simulink model "arduino_sw_harness"  (R2013b)
settings: Solver=FixedStepDiscrete  SolverMode=SingleTasking  StartTime=0.0  StopTime=10.0  FixedStep=0.1  RelTol=1e-3
libraries: arduinolib x3, simulink x1, sw_lib x1
settings Model: ExtModeTrigDuration=2  Creator=raarenst  LastModifiedBy=raarenst
settings OptimizationCC: OptimizeModelRefInitCode=on  LifeSpan=1
settings DebuggingCC: SolverPrmCheckMsg=none  ParameterPrecisionLossMsg=none
settings HardwareCC: ProdBitPerInt=16  ProdBitPerPointer=8  ProdIntDivRoundTo=Zero  ProdEndianess=LittleEndian  ProdWordSize=8  ProdHWDeviceType=Atmel->AVR
settings RTWCC: SystemTargetFile=realtime.tlc  GenerateMakefile=off  TemplateMakefile=realtime.tmf  Description=Run on Target Hardware  RTWVerbose=off  ProcessScript=realtime_make_rtw_hook
settings STFCustomTargetCC: TargetLibSuffix=.a  GenerateSampleERTMain=on  ERTCustomFileBanners=on  SupportNonInlinedSFcns=off  SupportVariableSizeSignals=on  MATLABClassNameForMDSCustomization=Simulink.SoftwareTarget.ERTCustomization  GRTInterface=off  SystemTargetFile=realtime.tlc
settings ERTTargetCC: CodeReplacementLibrary=ANSI_C  GenerateSampleERTMain=on  ParMdlRefBuildCompliant=off  CompOptLevelCompliant=off  ConcurrentExecutionCompliant=off  CombineOutputUpdateFcns=off  ERTFirstTimeCompliant=off  SupportContinuousTime=on  SupportVariableSizeSignals=on  ModelStepFunctionPrototypeControlCompliant=off  CPPClassGenCompliant=off  ExtModeTransport=3  ExtModeMexFile=ext_serial_win32_comm  ExtModeMexArgs=0 1 9600  InlinedParameterPlacement=NonHierarchical  ERTSrcFileBannerTemplate=realtime_code_template.cgt  ERTHdrFileBannerTemplate=realtime_code_template.cgt  ERTDataSrcFileTemplate=realtime_code_template.cgt  ERTDataHdrFileTemplate=realtime_code_template.cgt  ERTCustomFileTemplate=realtime_file_process.tlc
settings ConfigurationSet: Description=SimMechanics 2G

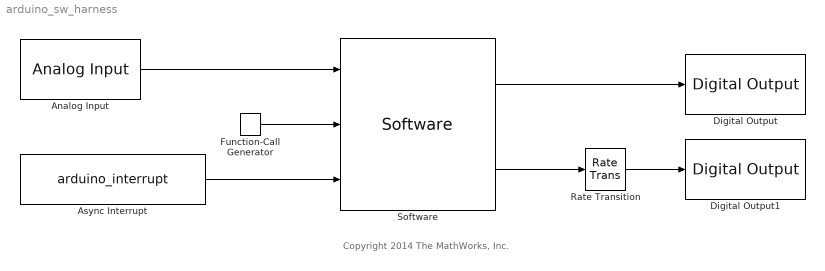
== system arduino_sw_harness ==
  note: Copyright 2014 The MathWorks, Inc.
  Analog Input : arduinolib/Analog Input  pinNumber=0  sampleTime=0.1
  Async Interrupt : S-Function  FunctionName=arduino_interrupt  Parameters=pin_number, int_number, int_mode, show_inputport  EnableBusSupport=off  mask(Arduino Interrupt Block){int_number=0, pin_number=2, int_mode=CHANGE, show_inputport=off}
      mask prompts: int_number "Interrupt number:"; pin_number "Pin number:"; int_mode "Mode:"; show_inputport "Enable simulation input:"
      mask help: Create Arduino interrupt service routine (ISR).
      mask init:
      | intNumStr = ['Int.', num2str(int_number)];
      | pinNumStr = ['pin ', num2str(pin_number)];
      | switch int_mode
      |     case 1
      |         pinModeStr = 'Mode: LOW';
      |     case 2
      |         pinModeStr = 'Mode: CHANGE';
      |     case 3
      |         pinModeStr ='Mode: RISING';
      |     case 4
      |         pinModeStr ='Mode: FALLING';
      |     otherwise
      |         pinModeStr = 'Mode: Error';
      | end
      | 
      | if ~show_inputport
      | 	% make the input port label disappear
      | 	pvalue = intNumStr;
      | 	pname = 'output';
      | else
      | 	pvalue = 'simIRQ';
      | 	pname = 'input';
      | end
      mask Help: eval('feval(''rtwprivate'',''rtwhelpview'',''rtw_async_interrupt_block'')');
      mask TypeOptions int_mode: LOW | CHANGE | RISING | FALLING
      mask Display:
      | color('blue');
      | text(0.55, 0.87, 'ARDUINO', 'horizontalAlignment','left');
      | color('black');
      | port_label('output',1, intNumStr);
      | port_label(pname,1,pvalue)
      | disp(pinNumStr);
      | text(0.5, 0.15, pinModeStr, 'horizontalAlignment', 'center');
  Digital Output : arduinolib/Digital Output  pinNumber=12
  Digital Output1 : arduinolib/Digital Output  pinNumber=13
  Function-Call Generator : simulink/Ports & Subsystems/Function-Call Generator  sample_time=0.1  numberOfIterations=1
  Rate Transition : RateTransition  Integrity=off
  Software : sw_lib/Software
  wires:
  Analog Input/1 -> Software/1
  Software/1 -> Digital Output/1
  Async Interrupt/1 -> Software/3
  Function-Call Generator/1 -> Software/2
  Software/2 -> Rate Transition/1
  Rate Transition/1 -> Digital Output1/1
